simulink model "linear_spacecraft_euler"  (R2015b)
settings: Solver=VariableStepAuto  StartTime=0.0  StopTime=10.0  RelTol=1e-3
values from neighbouring files (symbols this model uses):
  A = [zeros(3,3) eye(3);zeros(3,6)]    [main_reaction_wheels_design_v04.m]
  B = [zeros(3,3);diag([1/I_x 1/I_y 1/I_z])]    [main_nonlinear_spacecraft_euler.m]    (also in main_reaction_wheels_design_v04.m)
  C = eye(6)    [main_reaction_wheels_design_v04.m]
  D = zeros(6,3)    [main_reaction_wheels_design_v04.m]
  x_0 = [phi_0 ... (first row only)    [main_nonlinear_spacecraft_euler.m]    (also in main_nonlinear_spacecraft_quaternion.m = [epsilon_0; main_reaction_wheels_design_v04.m)
settings Model: Creator=Krunal's PC  LastModifiedBy=Krunal's PC

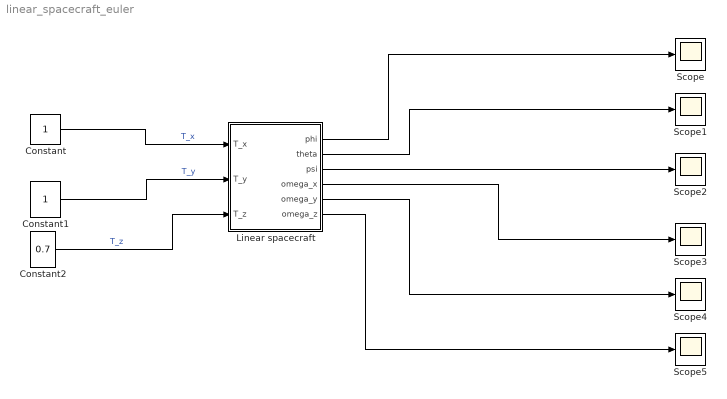
== system linear_spacecraft_euler ==
  Constant : Constant
  Constant1 : Constant
  Constant2 : Constant  Value=0.7
  Linear spacecraft : Subsystem
  Scope{,1..5} (6 alike) : Scope
  wires:
  Constant/1 -> Linear spacecraft/1(T_x)  "T_x"
  Constant1/1 -> Linear spacecraft/2(T_y)  "T_y"
  Constant2/1 -> Linear spacecraft/3(T_z)  "T_z"
  Linear spacecraft/1(phi) -> Scope/1
  Linear spacecraft/2(theta) -> Scope1/1
  Linear spacecraft/3(psi) -> Scope2/1
  Linear spacecraft/4(omega_x) -> Scope3/1
  Linear spacecraft/5(omega_y) -> Scope4/1
  Linear spacecraft/6(omega_z) -> Scope5/1

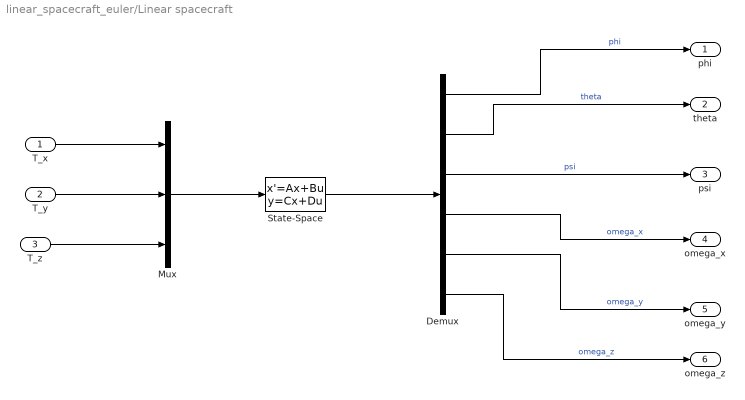
== system linear_spacecraft_euler/Linear spacecraft ==
  T_x : Inport
  T_y : Inport  Port=2
  T_z : Inport  Port=3
  Demux : Demux  Outputs=6
  Mux : Mux  Inputs=3
  State-Space : StateSpace  A=A  B=B  C=C  D=D  X0=x_0
  phi : Outport
  theta : Outport  Port=2
  psi : Outport  Port=3
  omega_x : Outport  Port=4
  omega_y : Outport  Port=5
  omega_z : Outport  Port=6
  wires:
  T_z/1 -> Mux/3
  State-Space/1 -> Demux/1
  T_y/1 -> Mux/2
  Demux/2 -> theta/1  "theta"
  Demux/6 -> omega_z/1  "omega_z"
  T_x/1 -> Mux/1
  Mux/1 -> State-Space/1
  Demux/5 -> omega_y/1  "omega_y"
  Demux/3 -> psi/1  "psi"
  Demux/1 -> phi/1  "phi"
  Demux/4 -> omega_x/1  "omega_x"
